simulink model "firBench"  (R2017b)
settings: Solver=FixedStepDiscrete  StartTime=0.0  StopTime=10000  FixedStep=0.1  RelTol=1e-3
libraries: dspsrcs4 x1
settings Model: Creator=cyarp  LastModifiedBy=cyarp

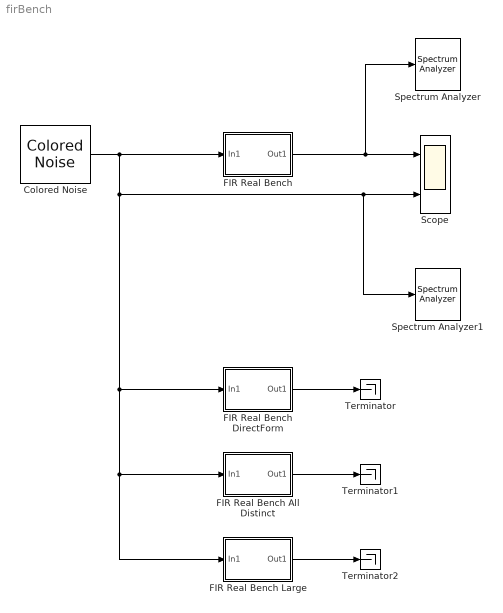
== system firBench ==
  Colored Noise : dspsrcs4/Colored Noise  Color=white  InverseFrequencyPower=1  NumChannels=1  OutputDataType=single  SamplesPerFrame=1  SampleTime=1  RandomStream=mt19937ar with seed  Seed=67  SimulateUsing=Interpreted execution
      settings: SourceProductName=DSP System Toolbox  SourceProductBaseCode=DS
  FIR Real Bench : Subsystem
  FIR Real Bench All Distinct : Subsystem
  FIR Real Bench DirectForm : Subsystem
  FIR Real Bench Large : Subsystem
  Scope : Scope  NumInputPorts=2
  Spectrum Analyzer : SpectrumAnalyzer
  Spectrum Analyzer1 : SpectrumAnalyzer
  Terminator : Terminator
  Terminator1 : Terminator
  Terminator2 : Terminator
  wires:
  FIR Real Bench/1(Out1) -> Spectrum Analyzer/1, Scope/1
  FIR Real Bench DirectForm/1(Out1) -> Terminator/1
  Colored Noise/1 -> FIR Real Bench/1(In1), FIR Real Bench Large/1(In1), FIR Real Bench All Distinct/1(In1), FIR Real Bench DirectForm/1(In1), Spectrum Analyzer1/1, Scope/2
  FIR Real Bench All Distinct/1(Out1) -> Terminator1/1
  FIR Real Bench Large/1(Out1) -> Terminator2/1

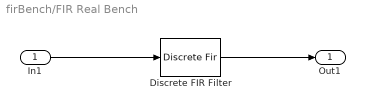
== system firBench/FIR Real Bench ==
  In1 : Inport
  Discrete FIR Filter : DiscreteFir  FilterStructure=Direct form transposed  Coefficients=[0.4, 0.2, 0.04, 0.1, 0.4, 0.2, 0.04, 0.1]  InitialStates=[0, 1, 0, 0, 0, 0, 0]
  Out1 : Outport
  wires:
  Discrete FIR Filter/1 -> Out1/1
  In1/1 -> Discrete FIR Filter/1

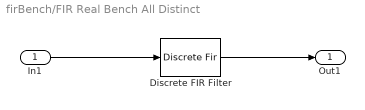
== system firBench/FIR Real Bench All Distinct ==
  In1 : Inport
  Discrete FIR Filter : DiscreteFir  FilterStructure=Direct form transposed  Coefficients=(1:1:8)+1
  Out1 : Outport
  wires:
  Discrete FIR Filter/1 -> Out1/1
  In1/1 -> Discrete FIR Filter/1

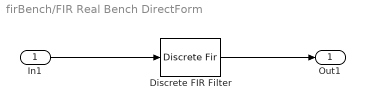
== system firBench/FIR Real Bench DirectForm ==
  In1 : Inport
  Discrete FIR Filter : DiscreteFir  Coefficients=[0.4, 0.2, 0.04, 0.1, 0.4, 0.2, 0.04, 0.1]  InitialStates=[0, 1, 0, 0, 0, 0, 0]
  Out1 : Outport
  wires:
  Discrete FIR Filter/1 -> Out1/1
  In1/1 -> Discrete FIR Filter/1

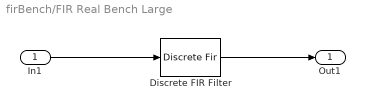
== system firBench/FIR Real Bench Large ==
  In1 : Inport
  Discrete FIR Filter : DiscreteFir  FilterStructure=Direct form transposed  Coefficients=(1:1:128)+1
  Out1 : Outport
  wires:
  Discrete FIR Filter/1 -> Out1/1
  In1/1 -> Discrete FIR Filter/1
